simulink model "rlWalkingBipedRobot_joint_test_v1"  (R2024b)
settings: Solver=ode23t  StartTime=0.0  StopTime=inf  RelTol=1e-2  EnableMultiTasking=on
undefined symbols (not defined in the file or in its folder): foot_z, height_plane, init_angs_R, init_height, joint_stiffness, max_torque, plane_x, plane_y, Tf, Ts, upper_leg_length, wx0, wy0, X, Y, Z
libraries: sm_lib x49, nesl_utility x29, walkingRobotUtils x6, simulink x2, rllib x1
(part 1 of 2)
settings Model: Creator=The MathWorks, Inc.  LastModifiedBy=joshp
settings SolverCC: ZeroCrossAlgorithm=Adaptive  AlgebraicLoopSolver=TrustRegion
settings DataIOCC: SaveOutput=off  SignalLogging=off  DSMLogging=off  SaveTime=off  OutputTimes=0:0.01:10
settings OptimizationCC: LifeSpan=inf
settings DebuggingCC: MaxConsecutiveZCsMsg=warning  IgnoredZcDiagnostic=none  UnconnectedInputMsg=warning  UnconnectedOutputMsg=warning  UnconnectedLineMsg=warning  AllowSymbolicDim=off  SFUnexpectedBacktrackingDiag=warning  SFNoUnconditionalDefaultTransitionDiag=warning  SFExecutionAtInitializationDiag=none  UnitsInconsistencyMsg=none  ArithmeticOperatorsInVariantConditions=warning
settings ModelReferenceCC: EnableRefExpFcnMdlSchedulingChecks=on
settings SFSimCC: SimUseLocalCustomCode=off  CustomCodeUndefinedFunction=UseInterfaceOnly
settings RTWCC: RTWUseLocalCustomCode=off  GPUComputeCapability=3.5
settings CodeAppCC: StateflowObjectComments=on
settings GRTTargetCC: TargetLangStandard=C89/C90 (ANSI)
settings ConfigComp: CovMetricSettings=dw  CovSaveCumulativeToWorkspaceVar=on  CovSaveSingleToWorkspaceVar=on  CovExternalEMLEnable=off  CovSFcnEnable=off
settings SimscapeCC: SimscapeNormalizeSystem=off  SimscapeLogOpenViewer=on  SimscapeLogLimitData=off  SimscapeLogDataHistory=10000
settings ConfigurationSet: Description=SimMechanics 2G
settings DiagnosticsConfigSet: SimMechanicsRigidlyBoundBlock=none
settings ExplorerConfigSet: InternalSimMechanicsExplorerSettings="<ExplorerConfiguration><canonicalview>default</canonicalview><AnimationSetting><BasePlaybackSpeed>1.0</BasePlaybackSpeed><PlaybackSpeedFactor>1.0</PlaybackSpeedFactor></AnimationSetting><TilePanel><TileInfo><Tiles Columns=\"1\" Count=\"1\" Rows=\"1\"><Column Weight=\"1\"/><Row Weight=\"1\"/><Tile Height=\"1\" Width=\"1\" X=\"0\" Y=\"0\"/></Tiles></TileInfo><SceneInfo><SceneViewer><BGColor><R>0.60000002384185791</R><G>0.60000002384185791</G><B>0.60000002384185791</B></BGColor><Camera><DoPerspective>off</DoPerspective><Position><X>7.18002534815406079</X><Y>-8.21011991112170847</Y><Z>8.33180938462712462</Z></Position><Center><X>1.10741005252516134</X><Y>-0.176829942633513204</Y><Z>0.646464709811595872</Z></Center><Up><X>-0.335329266167064488</X><Y>0.506481739462631531</Y><Z>0.79437430147428989</Z></Up><ViewLimDist>1</ViewLimDist><YLim>0.739205014828661411</YLim><XLim>1.12849377732657596</XLim></Camera></SceneViewer></SceneInfo></TilePanel><MechEditorPanel><Cameras/><GfxPanelCameraMap/><VideoCreator><PlaybackSpeedRatio>1.0</PlaybackSpeedRatio><FrameRate>30</FrameRate><VideoFormat>Motion JPEG AVI</VideoFormat><FrameSize>auto</FrameSize></VideoCreator></MechEditorPanel></ExplorerConfiguration>"

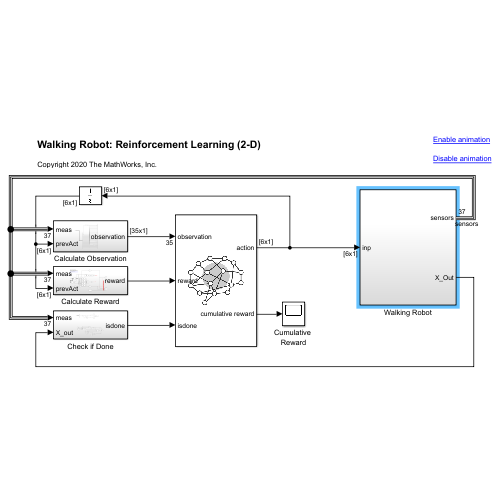
[thumbnail: Simulink's stored preview of the top-level diagram]
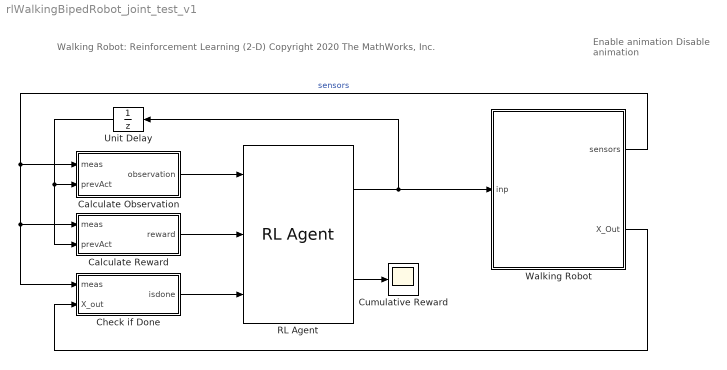
== system rlWalkingBipedRobot_joint_test_v1 ==
  note: Enable animation
      |
      | Disable animation
  note: Walking Robot: Reinforcement Learning (2-D)
      |
      | Copyright 2020 The MathWorks, Inc.
  Calculate Observation : Subsystem
  Calculate Reward : Subsystem
  Check if Done : Subsystem
  Cumulative Reward : Scope
  RL Agent : rllib/RL Agent  Agent=agent  ExternalActionAsInput=off  ProvideLastAction=off  ProvideCumRwd=on  TreatAsDirectFeedthrough=on  UseStrictObservationDataTypes=off
  Unit Delay : UnitDelay  SampleTime=-1  HasFrameUpgradeWarning=on
  Walking Robot : Subsystem
  wires:
  Walking Robot/1(sensors) -> Check if Done/1(meas), Calculate Reward/1(meas), Calculate Observation/1(meas)  "sensors"
  Calculate Reward/1(reward) -> RL Agent/2
  Calculate Observation/1(observation) -> RL Agent/1
  Check if Done/1(isdone) -> RL Agent/3
  RL Agent/2 -> Cumulative Reward/1
  Unit Delay/1 -> Calculate Reward/2(prevAct), Calculate Observation/2(prevAct)
  RL Agent/1 -> Walking Robot/1(inp), Unit Delay/1
  Walking Robot/2(X_Out) -> Check if Done/2(X_out)

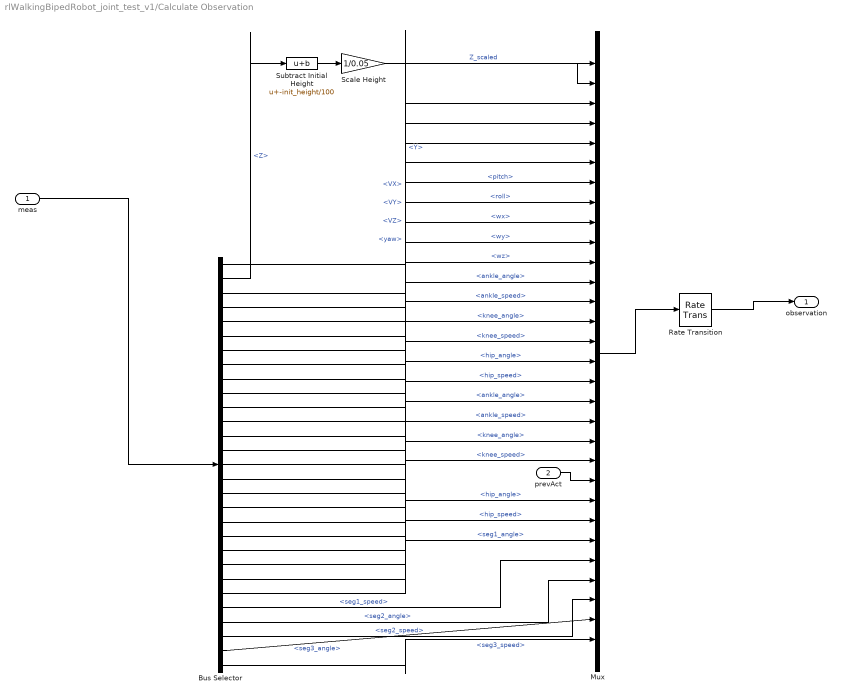
== system rlWalkingBipedRobot_joint_test_v1/Calculate Observation ==
  meas : Inport
  prevAct : Inport  Port=2
  Bus Selector : BusSelector  OutputSignals=Y,Z,VX,VY,VZ,yaw,pitch,roll,wx,wy,wz,measR.ankle_angle,measR.ankle_speed,measR.knee_angle,measR.knee_speed,measR.hip_angle,measR.hip_speed,measR.ankle_angle,measR.ankle_speed,measR.knee_angle,measR.knee_speed,measR.hip_angle,measR.hip_speed,measR.seg1_angle,measR.seg1_speed,measR.seg2_angle,measR.seg2_speed,measR.seg3_angle,measR.seg3_speed
  Mux : Mux  Inputs=30
  Rate Transition : RateTransition
  Scale Height : Gain  Gain=1/0.05
  Subtract Initial Height : Bias  Bias=-init_height/100  SaturateOnIntegerOverflow=off
  observation : Outport  VectorParamsAs1DForOutWhenUnconnected=off
  wires:
  meas/1 -> Bus Selector/1
  Mux/1 -> Rate Transition/1
  Rate Transition/1 -> observation/1
  prevAct/1 -> Mux/22
  Bus Selector/2 -> Subtract Initial Height/1  "<Z>"
  Subtract Initial Height/1 -> Scale Height/1
  Scale Height/1 -> Mux/2  "Z_scaled"
  Bus Selector/1 -> Mux/1  "<Y>"
  Bus Selector/4 -> Mux/4  "<VY>"
  Bus Selector/5 -> Mux/5  "<VZ>"
  Bus Selector/3 -> Mux/3  "<VX>"
  Bus Selector/6 -> Mux/6  "<yaw>"
  Bus Selector/7 -> Mux/7  "<pitch>"
  Bus Selector/8 -> Mux/8  "<roll>"
  Bus Selector/9 -> Mux/9  "<wx>"
  Bus Selector/10 -> Mux/10  "<wy>"
  Bus Selector/11 -> Mux/11  "<wz>"
  Bus Selector/12 -> Mux/12  "<ankle_angle>"
  Bus Selector/13 -> Mux/13  "<ankle_speed>"
  Bus Selector/14 -> Mux/14  "<knee_angle>"
  Bus Selector/15 -> Mux/15  "<knee_speed>"
  Bus Selector/16 -> Mux/16  "<hip_angle>"
  Bus Selector/17 -> Mux/17  "<hip_speed>"
  Bus Selector/18 -> Mux/18  "<ankle_angle>"
  Bus Selector/19 -> Mux/19  "<ankle_speed>"
  Bus Selector/20 -> Mux/20  "<knee_angle>"
  Bus Selector/21 -> Mux/21  "<knee_speed>"
  Bus Selector/22 -> Mux/23  "<hip_angle>"
  Bus Selector/23 -> Mux/24  "<hip_speed>"
  Bus Selector/24 -> Mux/25  "<seg1_angle>"
  Bus Selector/25 -> Mux/26  "<seg1_speed>"
  Bus Selector/26 -> Mux/27  "<seg2_angle>"
  Bus Selector/27 -> Mux/28  "<seg2_speed>"
  Bus Selector/28 -> Mux/29  "<seg3_angle>"
  Bus Selector/29 -> Mux/30  "<seg3_speed>"

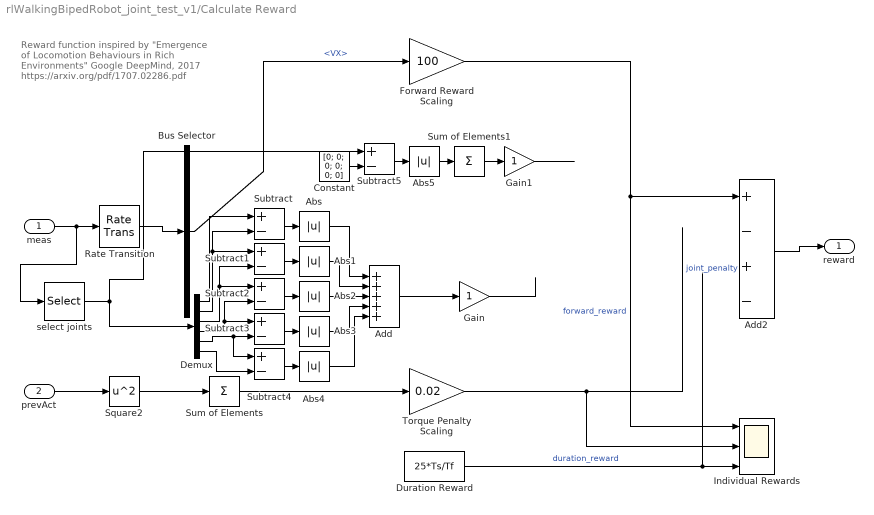
== system rlWalkingBipedRobot_joint_test_v1/Calculate Reward ==
  note: Reward function inspired by
      | "Emergence of Locomotion Behaviours in Rich Environments"
      | Google DeepMind, 2017
      | https://arxiv.org/pdf/1707.02286.pdf
  meas : Inport
  prevAct : Inport  Port=2
  Abs{,1..5} (6 alike) : Abs  SaturateOnIntegerOverflow=off
  Add : Sum  Inputs=+++++
  Add2 : Sum  Inputs=+-+-
  Bus Selector : BusSelector  OutputSignals=VX
  Constant : Constant  Value=[0; 0; 0; 0; 0; 0]  VectorParams1D=off
  Demux : Demux  Outputs=6
  Duration Reward : Constant  Value=25*Ts/Tf
  Forward Reward Scaling : Gain  Gain=100
  Gain : Gain
  Gain1 : Gain
  Individual Rewards : Scope  NumInputPorts=3
  Rate Transition : RateTransition  OutPortSampleTime=Ts
  Square2 : Math  Operator=square  SignedPower=on
  Subtract{,1..5} (6 alike) : Sum  Inputs=+-
  Sum of Elements : Sum  Inputs=+
  Sum of Elements1 : Sum  Inputs=+
  Torque Penalty Scaling : Gain  Gain=0.02
  select joints : Selector  InputPortWidth=37  IndexOptions=Index vector (dialog)  Indices=[3 6 9 12 15 18]  OutputSizes=1
  reward : Outport  VectorParamsAs1DForOutWhenUnconnected=off
  wires:
  meas/1 -> select joints/1, Rate Transition/1
  Rate Transition/1 -> Bus Selector/1
  Add2/1 -> reward/1
  Forward Reward Scaling/1 -> Individual Rewards/1, Add2/1  "forward_reward"
  Sum of Elements/1 -> Torque Penalty Scaling/1
  Bus Selector/1 -> Forward Reward Scaling/1  "<VX>"
  Duration Reward/1 -> Individual Rewards/3  "duration_reward"
  prevAct/1 -> Square2/1
  Square2/1 -> Sum of Elements/1
  Torque Penalty Scaling/1 -> Individual Rewards/2  "joint_penalty"
  select joints/1 -> Demux/1, Subtract5/1
  Demux/1 -> Subtract/1
  Demux/2 -> Subtract/2, Subtract1/1
  Demux/3 -> Subtract2/1, Subtract1/2
  Demux/4 -> Subtract3/1, Subtract2/2
  Demux/5 -> Subtract4/1, Subtract3/2
  Demux/6 -> Subtract4/2
  Subtract/1 -> Abs/1
  Subtract1/1 -> Abs1/1
  Subtract2/1 -> Abs2/1
  Subtract3/1 -> Abs3/1
  Subtract4/1 -> Abs4/1
  Abs/1 -> Add/1
  Abs1/1 -> Add/2
  Abs2/1 -> Add/3
  Abs3/1 -> Add/4
  Abs4/1 -> Add/5
  Add/1 -> Gain/1
  Gain/1 -> ?
  Constant/1 -> Subtract5/2
  Subtract5/1 -> Abs5/1
  Abs5/1 -> Sum of Elements1/1
  Sum of Elements1/1 -> Gain1/1
  Gain1/1 -> ?

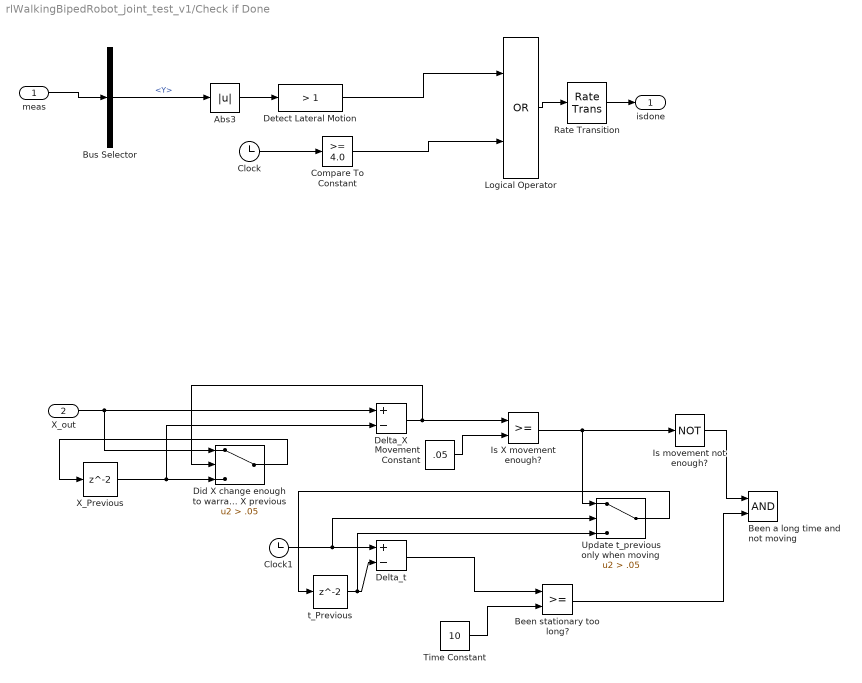
== system rlWalkingBipedRobot_joint_test_v1/Check if Done ==
  meas : Inport
  X_out : Inport  Port=2
  Abs3 : Abs  SaturateOnIntegerOverflow=off
  Been a long time and not moving : Logic  AllPortsSameDT=off  OutDataTypeStr=boolean
  Been stationary too long? : RelationalOperator  OutDataTypeStr=boolean  RndMeth=Simplest  InputSameDT=off
  Bus Selector : BusSelector  OutputSignals=Y
  Clock : Clock
  Clock1 : Clock
  Compare To Constant : simulink/Logic and Bit Operations/Compare To Constant  relop=>=  const=4.0  OutDataTypeStr=boolean
  Delta_X : Sum  Inputs=+-
  Delta_t : Sum  Inputs=+-
  Detect Lateral Motion : simulink/Logic and Bit Operations/Compare To Constant  relop=>  const=1  OutDataTypeStr=boolean
  Did X change enough to warrant an X previous : Switch  Criteria=u2 > Threshold  Threshold=.05  SaturateOnIntegerOverflow=off  InputSameDT=off
  Is X movement enough? : RelationalOperator  OutDataTypeStr=boolean  RndMeth=Simplest  InputSameDT=off
  Is movement not enough? : Logic  Operator=NOT  AllPortsSameDT=off  OutDataTypeStr=boolean
  Logical Operator : Logic  Operator=OR  AllPortsSameDT=off  OutDataTypeStr=boolean
  Movement Constant : Constant  Value=.05
  Rate Transition : RateTransition
  Time Constant : Constant  Value=10
  Update t_previous only when moving : Switch  Criteria=u2 > Threshold  Threshold=.05  SaturateOnIntegerOverflow=off  InputSameDT=off
  X_Previous : Delay
  t_Previous : Delay
  isdone : Outport  VectorParamsAs1DForOutWhenUnconnected=off
  wires:
  Logical Operator/1 -> Rate Transition/1
  meas/1 -> Bus Selector/1
  Rate Transition/1 -> isdone/1
  Bus Selector/1 -> Abs3/1  "<Y>"
  Detect Lateral Motion/1 -> Logical Operator/1
  Abs3/1 -> Detect Lateral Motion/1
  Clock/1 -> Compare To Constant/1
  Compare To Constant/1 -> Logical Operator/2
  Did X change enough to warrant an X previous/1 -> X_Previous/1
  Update t_previous only when moving/1 -> t_Previous/1
  Delta_t/1 -> Been stationary too long?/1
  Time Constant/1 -> Been stationary too long?/2
  Clock1/1 -> Update t_previous only when moving/2, Delta_t/1
  Been stationary too long?/1 -> Been a long time and not moving/2
  t_Previous/1 -> Update t_previous only when moving/3, Delta_t/2
  Is X movement enough?/1 -> Is movement not enough?/1, Update t_previous only when moving/1
  X_Previous/1 -> Did X change enough to warrant an X previous/3, Delta_X/2
  X_out/1 -> Did X change enough to warrant an X previous/1, Delta_X/1
  Delta_X/1 -> Did X change enough to warrant an X previous/2, Is X movement enough?/1
  Movement Constant/1 -> Is X movement enough?/2
  Is movement not enough?/1 -> Been a long time and not moving/1

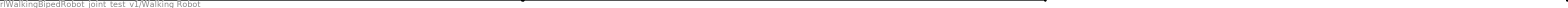
== system rlWalkingBipedRobot_joint_test_v1/Walking Robot ==
  note: masks_array
  note: 3 torques per leg
      | (ankle knee hip)
  inp : Inport
  6-DOF Joint : sm_lib/Joints/6-DOF Joint  JointMode=Normal  CompositeWrenchDir=FollowerOnBase  CompositeWrenchFrame=BaseFrame  SenseConstraintForce=off  SenseConstraintTorque=off  SenseTotalForce=off  SenseTotalTorque=off  PxPositionTargetSpecify=on  PxPositionTargetPriority=High  PxPositionTargetValue=0  PxPositionTargetValueUnits=m  PxVelocityTargetSpecify=on  PxVelocityTargetPriority=High  PxVelocityTargetValue=vx0  PxVelocityTargetValueUnits=m/s  PxEquilibriumPosition=0  PxEquilibriumPositionUnits=m  PxSpringStiffness=0  PxSpringStiffnessUnits=N/m  PxDampingCoefficient=world_damping  PxDampingCoefficientUnits=N/(m/s)  PxLowerLimitSpecify=off  PxLowerLimitBound=-1  PxLowerLimitBoundUnits=m  PxLowerLimitStiffness=1e6  PxLowerLimitStiffnessUnits=N/m  PxLowerLimitDamping=1e3  PxLowerLimitDampingUnits=N/(m/s)  PxLowerLimitTransitionRegionWidth=1e-4  PxLowerLimitTransitionRegionWidthUnits=m  PxUpperLimitSpecify=off  PxUpperLimitBound=1  PxUpperLimitBoundUnits=m  PxUpperLimitStiffness=1e6  PxUpperLimitStiffnessUnits=N/m  PxUpperLimitDamping=1e3  PxUpperLimitDampingUnits=N/(m/s)  PxUpperLimitTransitionRegionWidth=1e-4  PxUpperLimitTransitionRegionWidthUnits=m  PxTorqueActuationMode=NoTorque  PxMotionActuationMode=ComputedMotion  PxSensePosition=off  PxSenseVelocity=off  PxSenseAcceleration=off  PxSenseTorqueForce=off  PxSenseLowerLimitTorqueForce=off  PxSenseUpperLimitTorqueForce=off  PyPositionTargetSpecify=on  PyPositionTargetPriority=High  PyPositionTargetValue=0  PyPositionTargetValueUnits=m  PyVelocityTargetSpecify=on  PyVelocityTargetPriority=High  PyVelocityTargetValue=0  PyVelocityTargetValueUnits=m/s  PyEquilibriumPosition=0  PyEquilibriumPositionUnits=m  PySpringStiffness=0  PySpringStiffnessUnits=N/m  PyDampingCoefficient=world_damping  PyDampingCoefficientUnits=N/(m/s)  PyLowerLimitSpecify=off  PyLowerLimitBound=-1  PyLowerLimitBoundUnits=m  PyLowerLimitStiffness=1e6  PyLowerLimitStiffnessUnits=N/m  PyLowerLimitDamping=1e3  PyLowerLimitDampingUnits=N/(m/s)  PyLowerLimitTransitionRegionWidth=1e-4  PyLowerLimitTransitionRegionWidthUnits=m  PyUpperLimitSpecify=off  PyUpperLimitBound=1  PyUpperLimitBoundUnits=m  PyUpperLimitStiffness=1e6  PyUpperLimitStiffnessUnits=N/m  PyUpperLimitDamping=1e3  PyUpperLimitDampingUnits=N/(m/s)  PyUpperLimitTransitionRegionWidth=1e-4  PyUpperLimitTransitionRegionWidthUnits=m  PyTorqueActuationMode=NoTorque  PyMotionActuationMode=ComputedMotion  PySensePosition=off  PySenseVelocity=off  PySenseAcceleration=off  PySenseTorqueForce=off  PySenseLowerLimitTorqueForce=off  PySenseUpperLimitTorqueForce=off  PzPositionTargetSpecify=on  PzPositionTargetPriority=High  PzPositionTargetValue=init_height  PzPositionTargetValueUnits=cm  PzVelocityTargetSpecify=off  PzVelocityTargetPriority=High  PzVelocityTargetValue=0  PzVelocityTargetValueUnits=m/s  PzEquilibriumPosition=0  PzEquilibriumPositionUnits=m  PzSpringStiffness=0  PzSpringStiffnessUnits=N/m  PzDampingCoefficient=world_damping  PzDampingCoefficientUnits=N/(m/s)  PzLowerLimitSpecify=off  PzLowerLimitBound=-1  PzLowerLimitBoundUnits=m  PzLowerLimitStiffness=1e6  PzLowerLimitStiffnessUnits=N/m  PzLowerLimitDamping=1e3  PzLowerLimitDampingUnits=N/(m/s)  PzLowerLimitTransitionRegionWidth=1e-4  PzLowerLimitTransitionRegionWidthUnits=m  PzUpperLimitSpecify=off  PzUpperLimitBound=1  PzUpperLimitBoundUnits=m  PzUpperLimitStiffness=1e6  PzUpperLimitStiffnessUnits=N/m  PzUpperLimitDamping=1e3  PzUpperLimitDampingUnits=N/(m/s)  PzUpperLimitTransitionRegionWidth=1e-4  PzUpperLimitTransitionRegionWidthUnits=m  PzTorqueActuationMode=NoTorque  PzMotionActuationMode=ComputedMotion  PzSensePosition=off  PzSenseVelocity=off  PzSenseAcceleration=off  PzSenseTorqueForce=off  PzSenseLowerLimitTorqueForce=off  PzSenseUpperLimitTorqueForce=off  SphPositionTargetSpecify=on  SphPositionTargetPriority=High  SphPositionTargetRotationMethod=RotationSequence  SphPositionTargetFollAlignAxisA=+X  SphPositionTargetBaseAlignAxisA=+Y  SphPositionTargetFollAlignAxisB=+Y  SphPositionTargetBaseAlignAxisB=+Z  SphPositionTargetRotationStandardAxis=+Z  SphPositionTargetRotationAngle=0.0  SphPositionTargetRotationAngleUnits=deg  SphPositionTargetRotationArbitraryAxis=[0 0 1]  SphPositionTargetRotationSequenceAxes=FollowerAxes  SphPositionTargetRotationSequence=XYX  SphPositionTargetRotationSequenceAngles=[wx0 wy0 0]  SphPositionTargetRotationSequenceAnglesUnits=rad  SphPositionTargetRotationMatrix=eye(3)  SphPositionTargetQuaternion=[1 0 0 0]  SphVelocityTargetSpecify=off  SphVelocityTargetPriority=High  SphVelocityTargetValue=[0 0 0]  SphVelocityTargetValueUnits=deg/s  SphVelocityTargetInFollowerFrame=on  SphEqPosRotationMethod=None  SphEqPosFollAlignAxisA=+X  SphEqPosBaseAlignAxisA=+Y  SphEqPosFollAlignAxisB=+Y  SphEqPosBaseAlignAxisB=+Z  SphEqPosRotationStandardAxis=+Z  SphEqPosRotationAngle=0.0  SphEqPosRotationAngleUnits=deg  SphEqPosRotationArbitraryAxis=[0 0 1]  SphEqPosRotationSequenceAxes=FollowerAxes  SphEqPosRotationSequence=XYX  SphEqPosRotationSequenceAngles=[0 0 0]  SphEqPosRotationSequenceAnglesUnits=deg  SphEqPosRotationMatrix=[1 0 0; 0 1 0; 0 0 1]  SphEqPosQuaternion=[1 0 0 0]  SphSpringStiffness=0  SphSpringStiffnessUnits=N*m/deg  SphDampingCoefficient=world_rot_damping  SphDampingCoefficientUnits=N*m/(rad/s)  SphLowerLimitSpecify=off  SphLowerLimitBound=15  SphLowerLimitBoundUnits=deg  SphLowerLimitStiffness=1e4  SphLowerLimitStiffnessUnits=N*m/deg  SphLowerLimitDamping=10  SphLowerLimitDampingUnits=N*m/(deg/s)  SphLowerLimitTransitionRegionWidth=0.1  SphLowerLimitTransitionRegionWidthUnits=deg  SphUpperLimitSpecify=off  SphUpperLimitBound=45  SphUpperLimitBoundUnits=deg  SphUpperLimitStiffness=1e4  SphUpperLimitStiffnessUnits=N*m/deg  SphUpperLimitDamping=10  SphUpperLimitDampingUnits=N*m/(deg/s)  SphUpperLimitTransitionRegionWidth=0.1  SphUpperLimitTransitionRegionWidthUnits=deg  SphTorqueActuationMode=NoTorque  SphActuateTorqueX=off  SphActuateTorqueY=off  SphActuateTorqueZ=off  SphActuateTorque=off  SphActuationFrame=BaseFrame  SphSensePosition=off  SphSenseVelocityX=off  SphSenseVelocityY=off  SphSenseVelocityZ=off  SphSenseVelocity=off  SphSenseAccelerationX=off  SphSenseAccelerationY=off  SphSenseAccelerationZ=off  SphSenseAcceleration=off  SphSenseLowerLimitTorqueMag=off  SphSenseUpperLimitTorqueMag=off  SphSensingFrame=BaseFrame
  Actions : Scope
  Demux : Demux  Outputs=1
  Right Hip to Torso : sm_lib/Frames and Transforms/Rigid Transform  RotationMethod=None  FollAlignAxisA=+X  BaseAlignAxisA=+Y  FollAlignAxisB=+Y  BaseAlignAxisB=+Z  RotationStandardAxis=+Z  RotationAngle=0.0  RotationAngleUnits=deg  RotationArbitraryAxis=[0 0 1]  RotationSequenceAxes=FollowerAxes  RotationSequence=XYX  RotationSequenceAngles=[0 0 0]  RotationSequenceAnglesUnits=deg  RotationMatrix=[1 0 0; 0 1 0; 0 0 1]  Quaternion=[1 0 0 0]  TranslationMethod=Cartesian  TranslationCartesianOffset=[0 0 0]  TranslationCartesianOffsetUnits=cm  TranslationStandardAxis=+Z  TranslationStandardOffset=0  TranslationStandardOffsetUnits=cm  TranslationROffset=0  TranslationROffsetUnits=m  TranslationThetaOffset=0  TranslationThetaOffsetUnits=deg  TranslationZOffset=0  TranslationZOffsetUnits=m
  Robot Leg R : Subsystem
  Sensors : Subsystem
  Spatial Contact Force : sm_lib/Forces and Torques/Spatial Contact Force  NormalForceType=SmoothSpringDamper  NormalStiffness=contact_stiffness  NormalStiffnessUnits=N/m  NormalDamping=contact_damping  NormalDampingUnits=N/(m/s)  NormalTransitionRegionWidth=1e-4  NormalTransitionRegionWidthUnits=m  FrictionType=SmoothStickSlip  CoefficientOfStaticFriction=mu_s  CoefficientOfDynamicFriction=mu_k  FrictionalCriticalVelocity=mu_vth  FrictionalCriticalVelocityUnits=m/s  SenseContactSignal=off  SensePenetrationDepth=off  SenseSeparationDistance=off  SenseNormalForceMagnitude=on  SenseFrictionalForceMagnitude=on  SenseNormalVelocity=off  SenseTangentialVelocity=off  SenseContactBaseRotation=off  SenseContactBaseTranslation=off  SenseContactFollowerRotation=off  SenseContactFollowerTranslation=off  ZeroCrossDetectContactStartAndEnd=off
  Spherical Solid : sm_lib/Body Elements/Spherical Solid  SphereRadius=foot_z/2  SphereRadiusUnits=cm  ExportEntireGeometry=on  InertiaType=CalculateFromGeometry  BasedOnType=Mass  Density=1000  DensityUnits=kg/m^3  Mass=1  MassUnits=g  CenterOfMass=[0 0 0]  CenterOfMassUnits=m  MomentsOfInertia=[1 1 1]  MomentsOfInertiaUnits=kg*m^2  ProductsOfInertia=[0 0 0]  ProductsOfInertiaUnits=kg*m^2  GraphicType=FromGeometry  MarkerShape=Sphere  MarkerSize=10  GraphicVisPropType=SimpleVisualProperties  GraphicDiffuseColor=[0.5 0.5 0.5]  GraphicOpacity=1.0  GraphicSpecularColor=[0.5 0.5 0.5 1.0]  GraphicAmbientColor=[0.15 0.15 0.15 1.0]  GraphicEmissiveColor=[0.0 0.0 0.0 1.0]  GraphicShininess=75  DoExposeReferenceFrame=on  SerializedFrames=<Frames/>
  Spline : sm_lib/Curves and Surfaces/Spline  DataPoints=[0 0 0.025; 5 0 0.025]  DataPointsUnits=m  EndConditionType=Natural  GraphicType=FromGeometry  MarkerShape=Sphere  MarkerSize=10  GraphicVisPropType=SimpleVisualProperties  GraphicDiffuseColor=[0 0 0]  GraphicOpacity=1.0  GraphicSpecularColor=[0.5 0.5 0.5 1.0]  GraphicAmbientColor=[0.15 0.15 0.15 1.0]  GraphicEmissiveColor=[0.0 0.0 0.0 1.0]  GraphicShininess=75
  Torque Scaling : Gain  Gain=max_torque
  Torso : sm_lib/Body Elements/Brick Solid  BrickDimensions=[1 1 1]  BrickDimensionsUnits=cm  ExportEntireGeometry=off  InertiaType=CalculateFromGeometry  BasedOnType=Density  Density=density  DensityUnits=kg/m^3  Mass=1  MassUnits=kg  CenterOfMass=[0 0 0]  CenterOfMassUnits=m  MomentsOfInertia=[1 1 1]  MomentsOfInertiaUnits=kg*m^2  ProductsOfInertia=[1 1 1]  ProductsOfInertiaUnits=kg*m^2  GraphicType=FromGeometry  MarkerShape=Sphere  MarkerSize=10  GraphicVisPropType=SimpleVisualProperties  GraphicDiffuseColor=[0.5 0.5 0.5]  GraphicOpacity=1.0  GraphicSpecularColor=[0.5 0.5 0.5 1.0]  GraphicAmbientColor=[0.15 0.15 0.15 1.0]  GraphicEmissiveColor=[0.0 0.0 0.0 1.0]  GraphicShininess=75  DoExposeReferenceFrame=on  SerializedFrames=<Frames><Frame><Id>Frame1</Id><Value><Name>F1</Name><Origin><Source>CenterOfMassFrame</Source><FeatureName></FeatureName></Origin><PrimaryAxis><DefinedDirection>+Z</DefinedDirection><Source>ReferenceFrame</Source><SourceDirection>+Z</SourceDirection><FeatureName></FeatureName></PrimaryAxis><SecondaryAxis><DefinedDirection>+X</DefinedDirection><Source>ReferenceFrame</Source><SourceDirection>+X</SourceDirection><FeatureName></FeatureName></SecondaryAxis></Value></Frame></Frames>
  World and Ground : Subsystem
  sensors : Outport  VectorParamsAs1DForOutWhenUnconnected=off
  X_Out : Outport  Port=2
  wires:
  Robot Leg R/1(meas) -> Sensors/1(measR)
  Sensors/1(sensors) -> sensors/1
  Demux/1 -> Robot Leg R/1(torques), Actions/1  "right_torques"
  Torque Scaling/1 -> Demux/1
  inp/1 -> Torque Scaling/1
  Sensors/2(X_Out) -> X_Out/1
  connections:
  Spline/LConn1 -- Sensors/LConn1 -- 6-DOF Joint/LConn1 -- World and Ground/LConn1
  Robot Leg R/RConn2 -- Spatial Contact Force/LConn1 -- World and Ground/RConn1
  Robot Leg R/RConn1 -- Right Hip to Torso/RConn1
  6-DOF Joint/RConn1 -- Torso/RConn1 -- Sensors/RConn1 -- Right Hip to Torso/LConn1
  ?
  ?
  ?
  ?
  ?
  ?
  ?
  Spherical Solid/LConn1 -- Spatial Contact Force/RConn1
  Spherical Solid/RConn1 -- Torso/LConn1

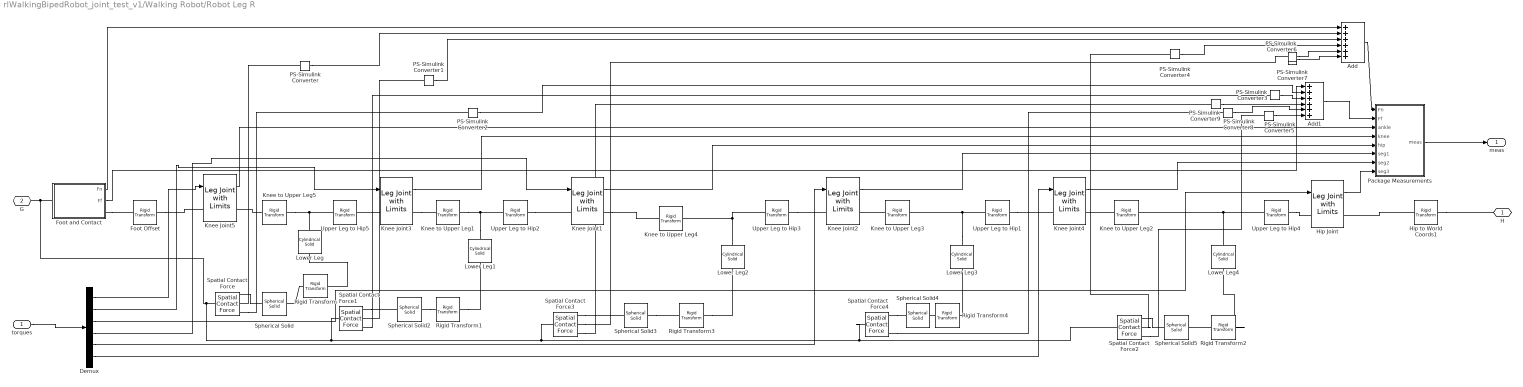
== system rlWalkingBipedRobot_joint_test_v1/Walking Robot/Robot Leg R ==
  torques : Inport
  Add : Sum  Inputs=++++++
  Add1 : Sum  Inputs=++++++
  Demux : Demux  Outputs=6
  Foot Offset : sm_lib/Frames and Transforms/Rigid Transform  RotationMethod=None  FollAlignAxisA=+X  BaseAlignAxisA=+Y  FollAlignAxisB=+Y  BaseAlignAxisB=+Z  RotationStandardAxis=+X  RotationAngle=-90  RotationAngleUnits=deg  RotationArbitraryAxis=[0 0 1]  RotationSequenceAxes=FollowerAxes  RotationSequence=XYX  RotationSequenceAngles=[0 0 0]  RotationSequenceAnglesUnits=deg  RotationMatrix=[1 0 0; 0 1 0; 0 0 1]  Quaternion=[1 0 0 0]  TranslationMethod=Cartesian  TranslationCartesianOffset=[0 0 0]  TranslationCartesianOffsetUnits=cm  TranslationStandardAxis=+Z  TranslationStandardOffset=0  TranslationStandardOffsetUnits=cm  TranslationROffset=0  TranslationROffsetUnits=m  TranslationThetaOffset=0  TranslationThetaOffsetUnits=deg  TranslationZOffset=0  TranslationZOffsetUnits=m
  Foot and Contact : Subsystem  AncestorBlock=walkingRobotUtils/Foot and Contact
  Hip Joint : walkingRobotUtils/Leg Joint with Limits  VariantControl=actuatorType == 2  k=joint_stiffness  d=joint_damping  initAngle=-init_angs_R(1)  eqAngle=0  upperLimit=pi/6  lowerLimit=-pi/6  jointLimitStiffness=joint_limit_stiffness  jointLimitDamping=joint_limit_damping
  Hip to World Coords1 : sm_lib/Frames and Transforms/Rigid Transform  RotationMethod=StandardAxis  FollAlignAxisA=+X  BaseAlignAxisA=+Y  FollAlignAxisB=+Y  BaseAlignAxisB=+Z  RotationStandardAxis=+X  RotationAngle=-90  RotationAngleUnits=deg  RotationArbitraryAxis=[0 0 1]  RotationSequenceAxes=FollowerAxes  RotationSequence=XYX  RotationSequenceAngles=[0 0 0]  RotationSequenceAnglesUnits=deg  RotationMatrix=[1 0 0; 0 1 0; 0 0 1]  Quaternion=[1 0 0 0]  TranslationMethod=None  TranslationCartesianOffset=[0 0 upper_leg_length/2]  TranslationCartesianOffsetUnits=cm  TranslationStandardAxis=+Z  TranslationStandardOffset=0  TranslationStandardOffsetUnits=cm  TranslationROffset=0  TranslationROffsetUnits=m  TranslationThetaOffset=0  TranslationThetaOffsetUnits=deg  TranslationZOffset=0  TranslationZOffsetUnits=m
  Knee Joint{1..5} (5 alike) : walkingRobotUtils/Leg Joint with Limits  VariantControl=actuatorType == 2  k=joint_stiffness  d=joint_damping  initAngle=init_angs_R(2)  eqAngle=0  upperLimit=pi/6  lowerLimit=-pi/6  jointLimitStiffness=joint_limit_stiffness  jointLimitDamping=joint_limit_damping
  Knee to Upper Leg{1..5} (5 alike) : sm_lib/Frames and Transforms/Rigid Transform  RotationMethod=StandardAxis  FollAlignAxisA=+X  BaseAlignAxisA=+Y  FollAlignAxisB=+Y  BaseAlignAxisB=+Z  RotationStandardAxis=+X  RotationAngle=-90  RotationAngleUnits=deg  RotationArbitraryAxis=[0 0 1]  RotationSequenceAxes=FollowerAxes  RotationSequence=XYX  RotationSequenceAngles=[0 0 0]  RotationSequenceAnglesUnits=deg  RotationMatrix=[1 0 0; 0 1 0; 0 0 1]  Quaternion=[1 0 0 0]  TranslationMethod=Cartesian  TranslationCartesianOffset=[0 upper_leg_length/2 0]  TranslationCartesianOffsetUnits=cm  TranslationStandardAxis=+Z  TranslationStandardOffset=0  TranslationStandardOffsetUnits=cm  TranslationROffset=0  TranslationROffsetUnits=m  TranslationThetaOffset=0  TranslationThetaOffsetUnits=deg  TranslationZOffset=0  TranslationZOffsetUnits=m
  Lower Leg : sm_lib/Body Elements/Cylindrical Solid  CylinderRadius=leg_radius  CylinderRadiusUnits=cm  CylinderLength=lower_leg_length  CylinderLengthUnits=cm  ExportEntireGeometry=off  InertiaType=CalculateFromGeometry  BasedOnType=Density  Density=density  DensityUnits=kg/m^3  Mass=1  MassUnits=kg  CenterOfMass=[0 0 0]  CenterOfMassUnits=m  MomentsOfInertia=[1 1 1]  MomentsOfInertiaUnits=kg*m^2  ProductsOfInertia=[1 1 1]  ProductsOfInertiaUnits=kg*m^2  GraphicType=FromGeometry  MarkerShape=Sphere  MarkerSize=10  GraphicVisPropType=SimpleVisualProperties  GraphicDiffuseColor=[1.0 0.2 0.2]  GraphicOpacity=1.0  GraphicSpecularColor=[0.5 0.5 0.5 1.0]  GraphicAmbientColor=[0.15 0.15 0.15 1.0]  GraphicEmissiveColor=[0.0 0.0 0.0 1.0]  GraphicShininess=75  DoExposeReferenceFrame=on  SerializedFrames=<Frames><Frame><Id>Frame1</Id><Value><Name>F1</Name><Origin><Source>GeometricFeature</Source><FeatureName>top surface</FeatureName></Origin><PrimaryAxis><DefinedDirection>+Z</DefinedDirection><Source>ReferenceFrame</Source><SourceDirection>+Z</SourceDirection><FeatureName></FeatureName></PrimaryAxis><SecondaryAxis><DefinedDirection>+X</DefinedDirection><Source>ReferenceFrame</Source><SourceDirection>+X</SourceDirection><FeatureName></FeatureName></SecondaryAxis></Value></Frame></Frames>
  Lower Leg1 : sm_lib/Body Elements/Cylindrical Solid  CylinderRadius=leg_radius  CylinderRadiusUnits=cm  CylinderLength=lower_leg_length  CylinderLengthUnits=cm  ExportEntireGeometry=off  InertiaType=CalculateFromGeometry  BasedOnType=Density  Density=density  DensityUnits=kg/m^3  Mass=1  MassUnits=kg  CenterOfMass=[0 0 0]  CenterOfMassUnits=m  MomentsOfInertia=[1 1 1]  MomentsOfInertiaUnits=kg*m^2  ProductsOfInertia=[1 1 1]  ProductsOfInertiaUnits=kg*m^2  GraphicType=FromGeometry  MarkerShape=Sphere  MarkerSize=10  GraphicVisPropType=SimpleVisualProperties  GraphicDiffuseColor=[1.0 1.0 0.0]  GraphicOpacity=1.0  GraphicSpecularColor=[0.5 0.5 0.5 1.0]  GraphicAmbientColor=[0.15 0.15 0.15 1.0]  GraphicEmissiveColor=[0.0 0.0 0.0 1.0]  GraphicShininess=75  DoExposeReferenceFrame=on  SerializedFrames=<Frames><Frame><Id>Frame1</Id><Value><Name>F1</Name><Origin><Source>GeometricFeature</Source><FeatureName>top surface</FeatureName></Origin><PrimaryAxis><DefinedDirection>+Z</DefinedDirection><Source>ReferenceFrame</Source><SourceDirection>+Z</SourceDirection><FeatureName></FeatureName></PrimaryAxis><SecondaryAxis><DefinedDirection>+X</DefinedDirection><Source>ReferenceFrame</Source><SourceDirection>+X</SourceDirection><FeatureName></FeatureName></SecondaryAxis></Value></Frame></Frames>
  Lower Leg2 : sm_lib/Body Elements/Cylindrical Solid  CylinderRadius=leg_radius  CylinderRadiusUnits=cm  CylinderLength=lower_leg_length  CylinderLengthUnits=cm  ExportEntireGeometry=off  InertiaType=CalculateFromGeometry  BasedOnType=Density  Density=density  DensityUnits=kg/m^3  Mass=1  MassUnits=kg  CenterOfMass=[0 0 0]  CenterOfMassUnits=m  MomentsOfInertia=[1 1 1]  MomentsOfInertiaUnits=kg*m^2  ProductsOfInertia=[1 1 1]  ProductsOfInertiaUnits=kg*m^2  GraphicType=FromGeometry  MarkerShape=Sphere  MarkerSize=10  GraphicVisPropType=SimpleVisualProperties  GraphicDiffuseColor=[0.0 1.0 0.0]  GraphicOpacity=1.0  GraphicSpecularColor=[0.5 0.5 0.5 1.0]  GraphicAmbientColor=[0.15 0.15 0.15 1.0]  GraphicEmissiveColor=[0.0 0.0 0.0 1.0]  GraphicShininess=75  DoExposeReferenceFrame=on  SerializedFrames=<Frames><Frame><Id>Frame1</Id><Value><Name>F1</Name><Origin><Source>GeometricFeature</Source><FeatureName>top surface</FeatureName></Origin><PrimaryAxis><DefinedDirection>+Z</DefinedDirection><Source>ReferenceFrame</Source><SourceDirection>+Z</SourceDirection><FeatureName></FeatureName></PrimaryAxis><SecondaryAxis><DefinedDirection>+X</DefinedDirection><Source>ReferenceFrame</Source><SourceDirection>+X</SourceDirection><FeatureName></FeatureName></SecondaryAxis></Value></Frame></Frames>
  Lower Leg3 : sm_lib/Body Elements/Cylindrical Solid  CylinderRadius=leg_radius  CylinderRadiusUnits=cm  CylinderLength=lower_leg_length  CylinderLengthUnits=cm  ExportEntireGeometry=off  InertiaType=CalculateFromGeometry  BasedOnType=Density  Density=density  DensityUnits=kg/m^3  Mass=1  MassUnits=kg  CenterOfMass=[0 0 0]  CenterOfMassUnits=m  MomentsOfInertia=[1 1 1]  MomentsOfInertiaUnits=kg*m^2  ProductsOfInertia=[1 1 1]  ProductsOfInertiaUnits=kg*m^2  GraphicType=FromGeometry  MarkerShape=Sphere  MarkerSize=10  GraphicVisPropType=SimpleVisualProperties  GraphicDiffuseColor=[0.0 0.8 1.0]  GraphicOpacity=1.0  GraphicSpecularColor=[0.5 0.5 0.5 1.0]  GraphicAmbientColor=[0.15 0.15 0.15 1.0]  GraphicEmissiveColor=[0.0 0.0 0.0 1.0]  GraphicShininess=75  DoExposeReferenceFrame=on  SerializedFrames=<Frames><Frame><Id>Frame1</Id><Value><Name>F1</Name><Origin><Source>GeometricFeature</Source><FeatureName>top surface</FeatureName></Origin><PrimaryAxis><DefinedDirection>+Z</DefinedDirection><Source>ReferenceFrame</Source><SourceDirection>+Z</SourceDirection><FeatureName></FeatureName></PrimaryAxis><SecondaryAxis><DefinedDirection>+X</DefinedDirection><Source>ReferenceFrame</Source><SourceDirection>+X</SourceDirection><FeatureName></FeatureName></SecondaryAxis></Value></Frame></Frames>
  Lower Leg4 : sm_lib/Body Elements/Cylindrical Solid  CylinderRadius=leg_radius  CylinderRadiusUnits=cm  CylinderLength=lower_leg_length  CylinderLengthUnits=cm  ExportEntireGeometry=off  InertiaType=CalculateFromGeometry  BasedOnType=Density  Density=density  DensityUnits=kg/m^3  Mass=1  MassUnits=kg  CenterOfMass=[0 0 0]  CenterOfMassUnits=m  MomentsOfInertia=[1 1 1]  MomentsOfInertiaUnits=kg*m^2  ProductsOfInertia=[1 1 1]  ProductsOfInertiaUnits=kg*m^2  GraphicType=FromGeometry  MarkerShape=Sphere  MarkerSize=10  GraphicVisPropType=SimpleVisualProperties  GraphicDiffuseColor=[0.6 0.0 0.6]  GraphicOpacity=1.0  GraphicSpecularColor=[0.5 0.5 0.5 1.0]  GraphicAmbientColor=[0.15 0.15 0.15 1.0]  GraphicEmissiveColor=[0.0 0.0 0.0 1.0]  GraphicShininess=75  DoExposeReferenceFrame=on  SerializedFrames=<Frames><Frame><Id>Frame1</Id><Value><Name>F1</Name><Origin><Source>GeometricFeature</Source><FeatureName>top surface</FeatureName></Origin><PrimaryAxis><DefinedDirection>+Z</DefinedDirection><Source>ReferenceFrame</Source><SourceDirection>+Z</SourceDirection><FeatureName></FeatureName></PrimaryAxis><SecondaryAxis><DefinedDirection>+X</DefinedDirection><Source>ReferenceFrame</Source><SourceDirection>+X</SourceDirection><FeatureName></FeatureName></SecondaryAxis></Value></Frame></Frames>
  PS-Simulink Converter{,1..9} (10 alike) : nesl_utility/PS-Simulink Converter  PhysicalDomain=network_engine_domain  SubClassName=ps_output  LeftPortType=input  RightPortType=output  PseudoPeriodic=off  Frequencies=[]  VectorFormat=inherit  Unit=inherit  AffineConversion=off
  Package Measurements : Subsystem  AncestorBlock="walkingRobotUtils/Package  Measurements 2D"
  Rigid Transform{,1,3..4} (4 alike) : sm_lib/Frames and Transforms/Rigid Transform  RotationMethod=None  FollAlignAxisA=+X  BaseAlignAxisA=+Y  FollAlignAxisB=+Y  BaseAlignAxisB=+Z  RotationStandardAxis=+Z  RotationAngle=0.0  RotationAngleUnits=deg  RotationArbitraryAxis=[0 0 1]  RotationSequenceAxes=FollowerAxes  RotationSequence=XYX  RotationSequenceAngles=[0 0 0]  RotationSequenceAnglesUnits=deg  RotationMatrix=[1 0 0; 0 1 0; 0 0 1]  Quaternion=[1 0 0 0]  TranslationMethod=None  TranslationCartesianOffset=[0 0 0]  TranslationCartesianOffsetUnits=m  TranslationStandardAxis=+Z  TranslationStandardOffset=0  TranslationStandardOffsetUnits=m  TranslationROffset=0  TranslationROffsetUnits=m  TranslationThetaOffset=0  TranslationThetaOffsetUnits=deg  TranslationZOffset=0  TranslationZOffsetUnits=m
  Rigid Transform2 : sm_lib/Frames and Transforms/Rigid Transform  RotationMethod=None  FollAlignAxisA=+X  BaseAlignAxisA=+Y  FollAlignAxisB=+Y  BaseAlignAxisB=+Z  RotationStandardAxis=+Z  RotationAngle=0.0  RotationAngleUnits=deg  RotationArbitraryAxis=[0 0 1]  RotationSequenceAxes=FollowerAxes  RotationSequence=XYX  RotationSequenceAngles=[0 0 0]  RotationSequenceAnglesUnits=deg  RotationMatrix=[1 0 0; 0 1 0; 0 0 1]  Quaternion=[1 0 0 0]  TranslationMethod=Cartesian  TranslationCartesianOffset=[0 0 0]  TranslationCartesianOffsetUnits=m  TranslationStandardAxis=+Z  TranslationStandardOffset=0  TranslationStandardOffsetUnits=m  TranslationROffset=0  TranslationROffsetUnits=m  TranslationThetaOffset=0  TranslationThetaOffsetUnits=deg  TranslationZOffset=0  TranslationZOffsetUnits=m
  Spatial Contact Force{,1..4} (5 alike) : sm_lib/Forces and Torques/Spatial Contact Force  NormalForceType=SmoothSpringDamper  NormalStiffness=contact_stiffness  NormalStiffnessUnits=N/m  NormalDamping=contact_damping  NormalDampingUnits=N/(m/s)  NormalTransitionRegionWidth=1e-4  NormalTransitionRegionWidthUnits=m  FrictionType=SmoothStickSlip  CoefficientOfStaticFriction=mu_s  CoefficientOfDynamicFriction=mu_k  FrictionalCriticalVelocity=mu_vth  FrictionalCriticalVelocityUnits=m/s  SenseContactSignal=off  SensePenetrationDepth=off  SenseSeparationDistance=off  SenseNormalForceMagnitude=on  SenseFrictionalForceMagnitude=on  SenseNormalVelocity=off  SenseTangentialVelocity=off  SenseContactBaseRotation=off  SenseContactBaseTranslation=off  SenseContactFollowerRotation=off  SenseContactFollowerTranslation=off  ZeroCrossDetectContactStartAndEnd=off
  Spherical Solid{,2..5} (5 alike) : sm_lib/Body Elements/Spherical Solid  SphereRadius=foot_z/2  SphereRadiusUnits=cm  ExportEntireGeometry=on  InertiaType=CalculateFromGeometry  BasedOnType=Mass  Density=1000  DensityUnits=kg/m^3  Mass=0  MassUnits=g  CenterOfMass=[0 0 0]  CenterOfMassUnits=m  MomentsOfInertia=[1 1 1]  MomentsOfInertiaUnits=kg*m^2  ProductsOfInertia=[0 0 0]  ProductsOfInertiaUnits=kg*m^2  GraphicType=FromGeometry  MarkerShape=Sphere  MarkerSize=10  GraphicVisPropType=SimpleVisualProperties  GraphicDiffuseColor=[0.5 0.5 0.5]  GraphicOpacity=1.0  GraphicSpecularColor=[0.5 0.5 0.5 1.0]  GraphicAmbientColor=[0.15 0.15 0.15 1.0]  GraphicEmissiveColor=[0.0 0.0 0.0 1.0]  GraphicShininess=75  DoExposeReferenceFrame=on  SerializedFrames=<Frames/>
  Upper Leg to Hip{1..5} (5 alike) : sm_lib/Frames and Transforms/Rigid Transform  RotationMethod=StandardAxis  FollAlignAxisA=+X  BaseAlignAxisA=+Y  FollAlignAxisB=+Y  BaseAlignAxisB=+Z  RotationStandardAxis=+X  RotationAngle=90  RotationAngleUnits=deg  RotationArbitraryAxis=[0 0 1]  RotationSequenceAxes=FollowerAxes  RotationSequence=XYX  RotationSequenceAngles=[0 0 0]  RotationSequenceAnglesUnits=deg  RotationMatrix=[1 0 0; 0 1 0; 0 0 1]  Quaternion=[1 0 0 0]  TranslationMethod=Cartesian  TranslationCartesianOffset=[0 0 upper_leg_length/2]  TranslationCartesianOffsetUnits=cm  TranslationStandardAxis=+Z  TranslationStandardOffset=0  TranslationStandardOffsetUnits=cm  TranslationROffset=0  TranslationROffsetUnits=m  TranslationThetaOffset=0  TranslationThetaOffsetUnits=deg  TranslationZOffset=0  TranslationZOffsetUnits=m
  H : PMIOPort  Side=Right
  G : PMIOPort  Port=2  Side=Right
  meas : Outport  VectorParamsAs1DForOutWhenUnconnected=off
  wires:
  Demux/3 -> Hip Joint/1
  Demux/2 -> Knee Joint3/1
  Demux/1 -> Knee Joint5/1
  Knee Joint5/1 -> Package Measurements/3(ankle)
  Knee Joint3/1 -> Package Measurements/4(knee)
  torques/1 -> Demux/1
  Package Measurements/1(meas) -> meas/1
  Demux/4 -> Knee Joint1/1
  Foot and Contact/1(Fn) -> Add/1
  PS-Simulink Converter/1 -> Add/2
  PS-Simulink Converter1/1 -> Add/3
  Add/1 -> Package Measurements/1(Fn)
  Foot and Contact/2(Ff) -> Add1/1
  PS-Simulink Converter2/1 -> Add1/2
  PS-Simulink Converter3/1 -> Add1/3
  Add1/1 -> Package Measurements/2(Ff)
  PS-Simulink Converter4/1 -> Add/4
  PS-Simulink Converter6/1 -> Add/6
  PS-Simulink Converter7/1 -> Add/5
  Demux/5 -> Knee Joint2/1
  Demux/6 -> Knee Joint4/1
  Hip Joint/1 -> Package Measurements/8(seg3)
  Knee Joint4/1 -> Package Measurements/7(seg2)
  Knee Joint2/1 -> Package Measurements/6(seg1)
  Knee Joint1/1 -> Package Measurements/5(hip)
  PS-Simulink Converter5/1 -> Add1/6
  PS-Simulink Converter9/1 -> Add1/4
  PS-Simulink Converter8/1 -> Add1/5
  connections:
  G/RConn1 -- Spatial Contact Force/LConn1 -- Spatial Contact Force4/LConn1 -- Spatial Contact Force2/LConn1 -- Spatial Contact Force3/LConn1 -- Spatial Contact Force1/LConn1 -- Foot and Contact/LConn1
  Foot and Contact/RConn1 -- Foot Offset/LConn1
  Hip to World Coords1/LConn1 -- Hip Joint/RConn1
  Knee to Upper Leg5/LConn1 -- Knee Joint5/RConn1
  Knee Joint3/RConn1 -- Knee to Upper Leg1/LConn1
  Lower Leg/RConn1 -- Knee to Upper Leg5/RConn1 -- Upper Leg to Hip5/LConn1
  Lower Leg1/RConn1 -- Upper Leg to Hip2/LConn1 -- Knee to Upper Leg1/RConn1
  Knee Joint3/LConn1 -- Upper Leg to Hip5/RConn1
  Hip to World Coords1/RConn1 -- H/RConn1
  Spatial Contact Force/RConn1 -- Spherical Solid/LConn1
  Lower Leg4/RConn1 -- Knee to Upper Leg2/RConn1 -- Upper Leg to Hip4/LConn1
  Upper Leg to Hip2/RConn1 -- Knee Joint1/LConn1
  Knee Joint1/RConn1 -- Knee to Upper Leg4/LConn1
  Upper Leg to Hip4/RConn1 -- Hip Joint/LConn1
  Spatial Contact Force1/RConn1 -- Spherical Solid2/LConn1
  Spherical Solid/RConn1 -- Rigid Transform/LConn1
  Lower Leg/LConn1 -- Rigid Transform/RConn1
  Spherical Solid2/RConn1 -- Rigid Transform1/LConn1
  Rigid Transform1/RConn1 -- Lower Leg1/LConn1
  Spatial Contact Force/RConn2 -- PS-Simulink Converter/LConn1
  PS-Simulink Converter1/LConn1 -- Spatial Contact Force1/RConn2
  Spatial Contact Force/RConn3 -- PS-Simulink Converter2/LConn1
  Spatial Contact Force1/RConn3 -- PS-Simulink Converter3/LConn1
  Rigid Transform2/LConn1 -- Spherical Solid5/RConn1
  Rigid Transform2/RConn1 -- Lower Leg4/LConn1
  Spatial Contact Force2/RConn1 -- Spherical Solid5/LConn1
  Spatial Contact Force2/RConn2 -- PS-Simulink Converter4/LConn1
  Spatial Contact Force2/RConn3 -- PS-Simulink Converter5/LConn1
  Upper Leg to Hip3/LConn1 -- Lower Leg2/RConn1 -- Knee to Upper Leg4/RConn1
  Lower Leg3/RConn1 -- Knee to Upper Leg3/RConn1 -- Upper Leg to Hip1/LConn1
  Rigid Transform3/RConn1 -- Lower Leg2/LConn1
  Spherical Solid3/RConn1 -- Rigid Transform3/LConn1
  Spatial Contact Force3/RConn1 -- Spherical Solid3/LConn1
  Spatial Contact Force4/RConn1 -- Spherical Solid4/LConn1
  Spherical Solid4/RConn1 -- Rigid Transform4/LConn1
  Rigid Transform4/RConn1 -- Lower Leg3/LConn1
  Upper Leg to Hip3/RConn1 -- Knee Joint2/LConn1
  Knee to Upper Leg3/LConn1 -- Knee Joint2/RConn1
  Upper Leg to Hip1/RConn1 -- Knee Joint4/LConn1
  Knee to Upper Leg2/LConn1 -- Knee Joint4/RConn1
  Spatial Contact Force3/RConn2 -- PS-Simulink Converter7/LConn1
  Spatial Contact Force4/RConn3 -- PS-Simulink Converter8/LConn1
  Spatial Contact Force3/RConn3 -- PS-Simulink Converter9/LConn1
  Foot Offset/RConn1 -- Knee Joint5/LConn1

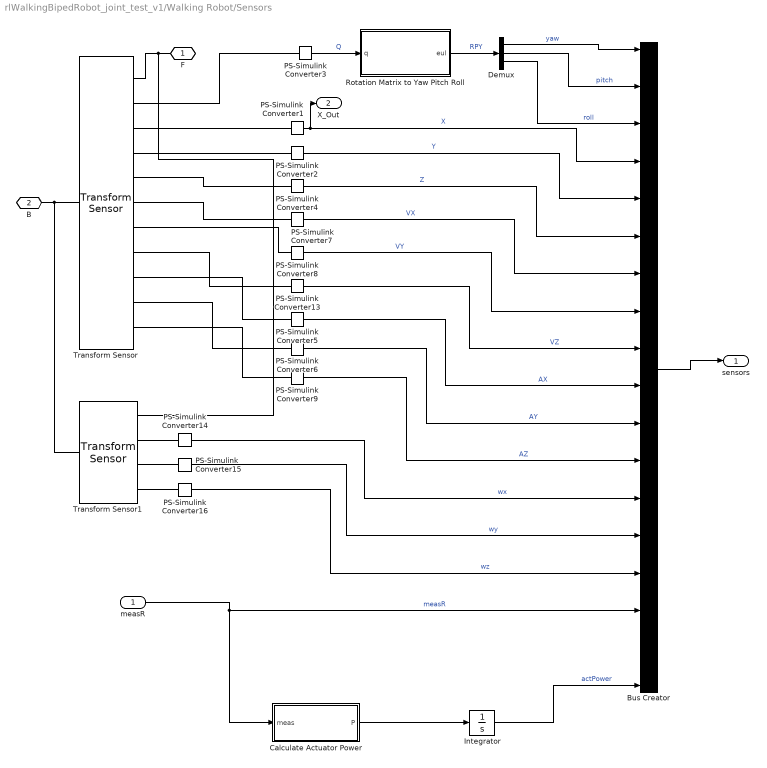
== system rlWalkingBipedRobot_joint_test_v1/Walking Robot/Sensors ==
  measR : Inport
  Bus Creator : BusCreator  Inputs=18
  Calculate Actuator Power : Subsystem
  Demux : Demux  Outputs=3
  Integrator : Integrator
  PS-Simulink Converter{1..9,13..16} (13 alike) : nesl_utility/PS-Simulink Converter  PhysicalDomain=network_engine_domain  SubClassName=ps_output  LeftPortType=input  RightPortType=output  PseudoPeriodic=off  Frequencies=[]  VectorFormat=1-D array  Unit=1  AffineConversion=off
  Rotation Matrix to Yaw Pitch Roll : MATLAB Function  TreatAsAtomicUnit=on
  Transform Sensor : sm_lib/Frames and Transforms/Transform Sensor  MeasurementFrame=World  RotationSequence=XYX  SenseAngle=off  SenseAxis=off  SenseQ=on  SenseR=off  SenseRotationSequence=off  SenseOmegaX=off  SenseOmegaY=off  SenseOmegaZ=off  SenseOmega=off  SenseQDot=off  SenseRDot=off  SenseRotationSequenceDot=off  SenseAlphaX=off  SenseAlphaY=off  SenseAlphaZ=off  SenseAlpha=off  SenseQDDot=off  SenseRDDot=off  SenseX=on  SenseY=on  SenseZ=on  SenseXYZ=off  SenseRad=off  SenseAzim=off  SenseDist=off  SenseInc=off  SenseXDot=on  SenseYDot=on  SenseZDot=on  SenseXYZDot=off  SenseRadDot=off  SenseAzimDot=off  SenseDistDot=off  SenseIncDot=off  SenseXDDot=on  SenseYDDot=on  SenseZDDot=on  SenseXYZDDot=off  SenseRadDDot=off  SenseAzimDDot=off  SenseDistDDot=off  SenseIncDDot=off
  Transform Sensor1 : sm_lib/Frames and Transforms/Transform Sensor  MeasurementFrame=NonRotatingFollower  RotationSequence=XYX  SenseAngle=off  SenseAxis=off  SenseQ=off  SenseR=off  SenseRotationSequence=off  SenseOmegaX=on  SenseOmegaY=on  SenseOmegaZ=on  SenseOmega=off  SenseQDot=off  SenseRDot=off  SenseRotationSequenceDot=off  SenseAlphaX=off  SenseAlphaY=off  SenseAlphaZ=off  SenseAlpha=off  SenseQDDot=off  SenseRDDot=off  SenseX=off  SenseY=off  SenseZ=off  SenseXYZ=off  SenseRad=off  SenseAzim=off  SenseDist=off  SenseInc=off  SenseXDot=off  SenseYDot=off  SenseZDot=off  SenseXYZDot=off  SenseRadDot=off  SenseAzimDot=off  SenseDistDot=off  SenseIncDot=off  SenseXDDot=off  SenseYDDot=off  SenseZDDot=off  SenseXYZDDot=off  SenseRadDDot=off  SenseAzimDDot=off  SenseDistDDot=off  SenseIncDDot=off
  F : PMIOPort  Side=Right
  B : PMIOPort  Port=2  Side=Left
  sensors : Outport  VectorParamsAs1DForOutWhenUnconnected=off
  X_Out : Outport  Port=2
  wires:
  PS-Simulink Converter2/1 -> Bus Creator/5  "Y"
  PS-Simulink Converter4/1 -> Bus Creator/6  "Z"
  PS-Simulink Converter5/1 -> Bus Creator/10  "AX"
  Bus Creator/1 -> sensors/1
  PS-Simulink Converter3/1 -> Rotation Matrix to Yaw Pitch Roll/1(q)  "Q"
  PS-Simulink Converter1/1 -> X_Out/1, Bus Creator/4  "X"
  PS-Simulink Converter6/1 -> Bus Creator/11  "AY"
  PS-Simulink Converter7/1 -> Bus Creator/7  "VX"
  PS-Simulink Converter8/1 -> Bus Creator/8  "VY"
  PS-Simulink Converter9/1 -> Bus Creator/12  "AZ"
  PS-Simulink Converter13/1 -> Bus Creator/9  "VZ"
  Rotation Matrix to Yaw Pitch Roll/1(eul) -> Demux/1  "RPY"
  Demux/3 -> Bus Creator/3  "roll"
  Demux/2 -> Bus Creator/2  "pitch"
  Demux/1 -> Bus Creator/1  "yaw"
  PS-Simulink Converter14/1 -> Bus Creator/13  "wx"
  PS-Simulink Converter15/1 -> Bus Creator/14  "wy"
  PS-Simulink Converter16/1 -> Bus Creator/15  "wz"
  measR/1 -> Calculate Actuator Power/1(meas), Bus Creator/16  "measR"
  Integrator/1 -> Bus Creator/18  "actPower"
  Calculate Actuator Power/1(P) -> Integrator/1
  connections:
  PS-Simulink Converter1/LConn1 -- Transform Sensor/RConn3
  PS-Simulink Converter3/LConn1 -- Transform Sensor/RConn2
  Transform Sensor/RConn1 -- Transform Sensor1/RConn1 -- F/RConn1
  Transform Sensor/RConn5 -- PS-Simulink Converter4/LConn1
  Transform Sensor/RConn4 -- PS-Simulink Converter2/LConn1
  Transform Sensor/LConn1 -- Transform Sensor1/LConn1 -- B/RConn1
  PS-Simulink Converter7/LConn1 -- Transform Sensor/RConn6
  PS-Simulink Converter14/LConn1 -- Transform Sensor1/RConn2
  PS-Simulink Converter15/LConn1 -- Transform Sensor1/RConn3
  Transform Sensor1/RConn4 -- PS-Simulink Converter16/LConn1
  Transform Sensor/RConn7 -- PS-Simulink Converter8/LConn1
  PS-Simulink Converter13/LConn1 -- Transform Sensor/RConn8
  PS-Simulink Converter5/LConn1 -- Transform Sensor/RConn9
  Transform Sensor/RConn10 -- PS-Simulink Converter6/LConn1
  PS-Simulink Converter9/LConn1 -- Transform Sensor/RConn11

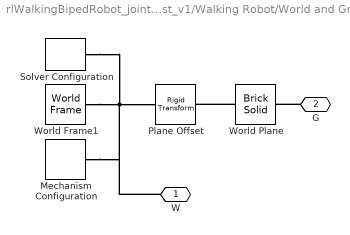
== system rlWalkingBipedRobot_joint_test_v1/Walking Robot/World and Ground ==
  Mechanism Configuration : sm_lib/Utilities/Mechanism Configuration  UniformGravity=Constant  GravityVector=[0 0 -9.80665]  GravityVectorUnits=m/s^2  LinearizationDelta=0.001  JointModeTransitionNonlinearIterations=2
  Plane Offset : sm_lib/Frames and Transforms/Rigid Transform  RotationMethod=None  FollAlignAxisA=+X  BaseAlignAxisA=+Y  FollAlignAxisB=+Y  BaseAlignAxisB=+Z  RotationStandardAxis=+Z  RotationAngle=0.0  RotationAngleUnits=deg  RotationArbitraryAxis=[0 0 1]  RotationSequenceAxes=FollowerAxes  RotationSequence=XYX  RotationSequenceAngles=[0 0 0]  RotationSequenceAnglesUnits=deg  RotationMatrix=[1 0 0; 0 1 0; 0 0 1]  Quaternion=[1 0 0 0]  TranslationMethod=StandardAxis  TranslationCartesianOffset=[0 0 0]  TranslationCartesianOffsetUnits=m  TranslationStandardAxis=-Z  TranslationStandardOffset=height_plane/2  TranslationStandardOffsetUnits=m  TranslationROffset=0  TranslationROffsetUnits=m  TranslationThetaOffset=0  TranslationThetaOffsetUnits=deg  TranslationZOffset=0  TranslationZOffsetUnits=m
  Solver Configuration : nesl_utility/Solver Configuration  PhysicalDomain=network_engine_domain  SubClassName=solver  LeftPortType=input  RightPortType=generic  Tones=[]  Harmonics=[]  SimulateNoise=off  Profile=off  UseLocalSampling=off  EnableSwitchedLinearOptims=on  FrequencyDomain=off  UseCCode=off  RelTol=0.001  AbsTol=1e-06  MinStep=1e-09  ToWorkspace=off  RevertToSquareIcSolve=off  NumHomotopyIterations=100  PhasorMode=off  PhasorModeNumHarmonics=1  ConsistencySolver=NEWTON_FTOL  IndexReductionMethod=DerivativeReplacement  DoDC=off  ResidualTolerance=1e-09  ConsistencyTolSource=GLOBAL  ConsistencyAbsTol=0.001  ConsistencyRelTol=0.001  ConsistencyTolFactor=0.001  UseLocalSolver=off  LocalSolverChoice=NE_TRAPEZOIDAL_ADVANCER  ResolveIndetEquations=on  FunctionEvalNumThread=1  LocalSolverSampleTime=Ts  DoFixedCost=off  MaxNonlinIter=3  MaxModeIter=2  ComputeImpulses=off  ImpulseIterations=2  LinearAlgebra=Sparse  LinearAlgebraNumThread=0  EquationFormulation=NE_TIME_EF  DelaysMemoryBudget=1024  AutomaticFiltering=on  FilteringTimeConstant=0.001  PartitionStorageMethod=AS_NEEDED  PartitionMemoryBudget=1024  PartitionMethod=FAST  MultibodyUseLocalSolver=off  MultibodyLocalSolverChoice=ODE1  MultibodyLocalSolverSampleTime=0.001
  World Frame1 : sm_lib/Frames and Transforms/World Frame
  World Plane : sm_lib/Body Elements/Brick Solid  BrickDimensions="[plane_x plane_y  height_plane]"  BrickDimensionsUnits=m  ExportEntireGeometry=on  InertiaType=CalculateFromGeometry  BasedOnType=Density  Density=density  DensityUnits=kg/(m^3)  Mass=1  MassUnits=kg  CenterOfMass=[0 0 0]  CenterOfMassUnits=m  MomentsOfInertia=[1 1 1]  MomentsOfInertiaUnits=kg*m^2  ProductsOfInertia=[0 0 0]  ProductsOfInertiaUnits=kg*m^2  GraphicType=FromGeometry  MarkerShape=Sphere  MarkerSize=10  GraphicVisPropType=SimpleVisualProperties  GraphicDiffuseColor=[1.0 1.0 0.8]  GraphicOpacity=0.5  GraphicSpecularColor=[0.5 0.5 0.5 1.0]  GraphicAmbientColor=[0.15 0.15 0.15 1.0]  GraphicEmissiveColor=[0.0 0.0 0.0 1.0]  GraphicShininess=75  DoExposeReferenceFrame=on  SerializedFrames=<Frames/>
  W : PMIOPort  Side=Left
  G : PMIOPort  Port=2  Side=Right
  connections:
  G/RConn1 -- World Plane/LConn1
  World Plane/RConn1 -- Plane Offset/RConn1
  Solver Configuration/RConn1 -- Plane Offset/LConn1 -- Mechanism Configuration/RConn1 -- W/RConn1 -- World Frame1/RConn1
